simulink model "stateflow_truthtable"  (R2015b)
settings: Solver=VariableStepAuto  StartTime=0.0  StopTime=10.0  RelTol=1e-3
settings Model: Creator=ladmin  LastModifiedBy=ladmin

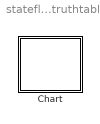
== system stateflow_truthtable ==
  Chart : Stateflow chart  TreatAsAtomicUnit=on

== matlab function stateflow_truthtable/Chart ==
function t1
